simulink model "LagrangeDynamics"  (R2015a)
settings: Solver=ode5  StartTime=0.0  StopTime=10  FixedStep=0.01  RelTol=1e-3
settings Model: Creator=Fares  LastModifiedBy=Fares

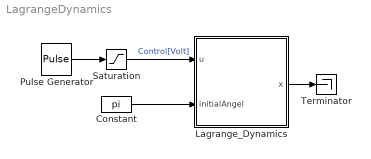
== system LagrangeDynamics ==
  Constant : Constant  Value=pi
  Lagrange_Dynamics : Subsystem  mask{mp=0.95 + 0.025, mc=1.12, l=0.033245968, I=0.013935418, fp=0.000107443, MF=9.4, g=9.81}
      mask prompts: mp "Pedulum mass [kg]"; mc "Cart mass [kg]"; l "Distance from the base to the system CoM [m]"; I "Pendulum of moment of inertia [kg*m2]"; fp "Rotational friction [N ms/rad]"; MF "Maximum Control force [N]"; g "Gravitational acceleration [m/s2]"
      mask init:
      | vf = MF/2.5;
      | M = mc + mp;
      | It = I + mp*l^2;
  Pulse Generator : DiscretePulseGenerator  PulseType=Time based  Period=100  PulseWidth=0.5
  Saturation : Saturate  UpperLimit=2.5  LowerLimit=-2.5
  Terminator : Terminator
  wires:
  Saturation/1 -> Lagrange_Dynamics/1(u)  "Control[Volt]"
  Pulse Generator/1 -> Saturation/1
  Constant/1 -> Lagrange_Dynamics/2(initialAngel)
  Lagrange_Dynamics/1(x) -> Terminator/1

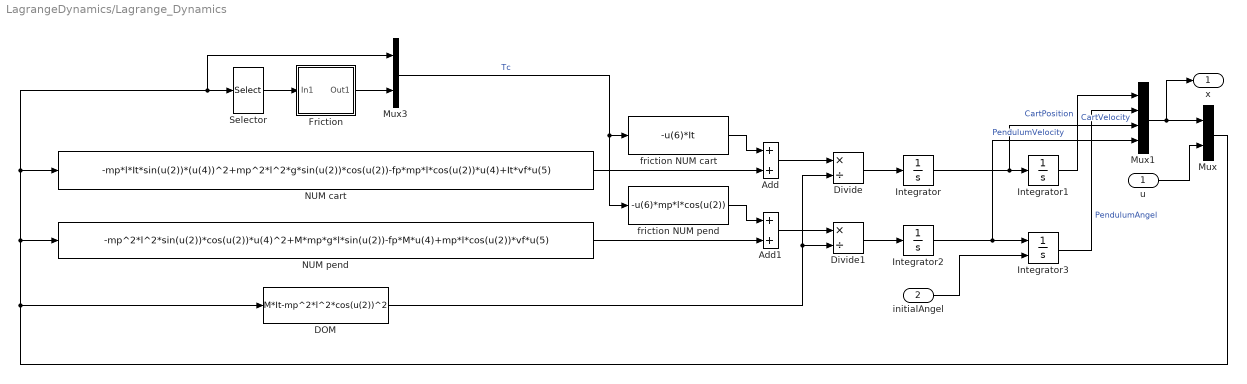
== system LagrangeDynamics/Lagrange_Dynamics ==
  u : Inport
  initialAngel : Inport  Port=2
  Add : Sum
  Add1 : Sum
  "DOM " : Fcn  Expr=M*It-mp^2*l^2*cos(u(2))^2
  Divide : Product  Inputs=*/
  Divide1 : Product  Inputs=*/
  Friction : Subsystem  mask{FS=2.53165, FC=2.28133, DZcv=0.00793711, Xc=0.9, Yc=2.3}
      mask prompts: FS "Static friction [N]"; FC "Coulombic friction [N]"; DZcv "Minimum cart velocity [rad/s]"; Xc "Cart velocity - beginning of the linear dependence zone [m/s]"; Yc "Friction value for Xc point [N]"
      mask init:
      | small = DZcv;
      mask Display: plot([-4 4],[0 0],[-3.8 -2.4 -1.8 -1.2 -0.6 -0.2 0 0.2 0.6 1.2 1.8 2.4 3.8],[-1.4 -1 -1.1 -1.3 -1.6 -2 0 2 1.6 1.3 1.1 1 1.4]);
  Integrator : Integrator
  Integrator1 : Integrator
  Integrator2 : Integrator
  Integrator3 : Integrator  InitialConditionSource=external  InitialCondition=pi
  Mux : Mux  Inputs=2
  Mux1 : Mux
  Mux3 : Mux  Inputs=2
  "NUM cart " : Fcn  Expr=-mp*l*It*sin(u(2))*(u(4))^2+mp^2*l^2*g*sin(u(2))*cos(u(2))-fp*mp*l*cos(u(2))*u(4)+It*vf*u(5)
  NUM pend : Fcn  Expr=-mp^2*l^2*sin(u(2))*cos(u(2))*u(4)^2+M*mp*g*l*sin(u(2))-fp*M*u(4)+mp*l*cos(u(2))*vf*u(5)
  Selector : Selector  InputPortWidth=5  Indices=[3]
  friction NUM cart : Fcn  Expr=-u(6)*It
  friction NUM pend : Fcn  Expr=-u(6)*mp*l*cos(u(2))
  x : Outport
  wires:
  "DOM "/1 -> Divide/2, Divide1/2
  Mux/1 -> Mux3/1, Selector/1, "NUM cart "/1, NUM pend/1, "DOM "/1
  Divide/1 -> Integrator/1
  Integrator2/1 -> Mux1/4, Integrator3/1  "PendulumVelocity"
  u/1 -> Mux/2
  Divide1/1 -> Integrator2/1
  Integrator1/1 -> Mux1/1  "CartPosition"
  Integrator3/1 -> Mux1/2  "PendulumAngel"
  initialAngel/1 -> Integrator3/2
  Integrator/1 -> Mux1/3, Integrator1/1  "CartVelocity"
  Mux1/1 -> x/1, Mux/1
  Selector/1 -> Friction/1(In1)
  "NUM cart "/1 -> Add/2
  NUM pend/1 -> Add1/2
  friction NUM cart/1 -> Add/1
  friction NUM pend/1 -> Add1/1
  Friction/1(Out1) -> Mux3/2
  Mux3/1 -> friction NUM pend/1, friction NUM cart/1  "Tc"
  Add/1 -> Divide/1
  Add1/1 -> Divide1/1

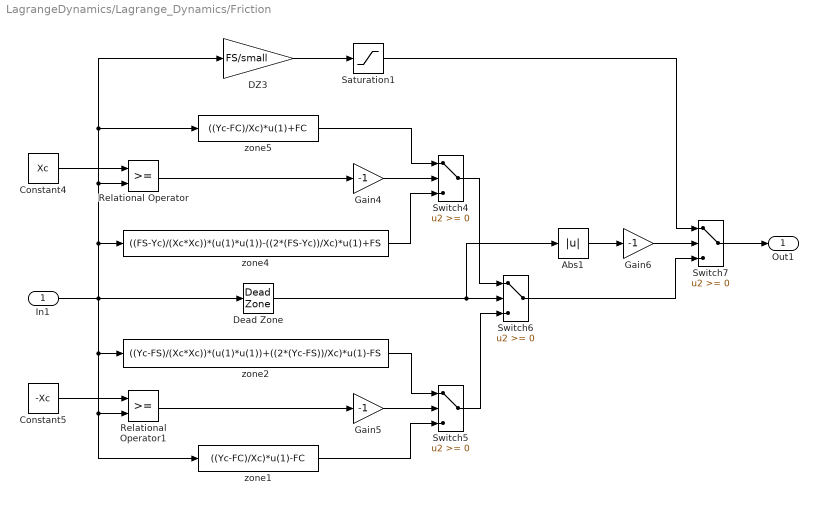
== system LagrangeDynamics/Lagrange_Dynamics/Friction ==
  In1 : Inport
  Abs1 : Abs
  Constant4 : Constant  Value=Xc
  Constant5 : Constant  Value=-Xc
  DZ3 : Gain  Gain=FS/small
  Dead Zone : DeadZone  LowerValue=-DZcv  UpperValue=DZcv  SaturateOnIntegerOverflow=on
  Gain4 : Gain  Gain=-1
  Gain5 : Gain  Gain=-1
  Gain6 : Gain  Gain=-1
  Relational Operator : RelationalOperator  OutDataTypeStr=boolean
  Relational Operator1 : RelationalOperator  OutDataTypeStr=boolean
  Saturation1 : Saturate  UpperLimit=FS  LowerLimit=-FS
  Switch{4..7} (4 alike) : Switch
  zone1 : Fcn  Expr=((Yc-FC)/Xc)*u(1)-FC
  zone2 : Fcn  Expr=((Yc-FS)/(Xc*Xc))*(u(1)*u(1))+((2*(Yc-FS))/Xc)*u(1)-FS
  zone4 : Fcn  Expr=((FS-Yc)/(Xc*Xc))*(u(1)*u(1))-((2*(FS-Yc))/Xc)*u(1)+FS
  zone5 : Fcn  Expr=((Yc-FC)/Xc)*u(1)+FC
  Out1 : Outport
  wires:
  Gain4/1 -> Switch4/2
  Dead Zone/1 -> Abs1/1, Switch6/2
  Gain5/1 -> Switch5/2
  Relational Operator/1 -> Gain4/1
  Constant5/1 -> Relational Operator1/1
  Relational Operator1/1 -> Gain5/1
  Abs1/1 -> Gain6/1
  DZ3/1 -> Saturation1/1
  Switch6/1 -> Switch7/3
  Switch4/1 -> Switch6/1
  zone2/1 -> Switch5/1
  Gain6/1 -> Switch7/2
  zone4/1 -> Switch4/3
  Switch7/1 -> Out1/1
  In1/1 -> zone1/1, Relational Operator1/2, zone2/1, DZ3/1, zone5/1, Relational Operator/2, zone4/1, Dead Zone/1
  Saturation1/1 -> Switch7/1
  zone5/1 -> Switch4/1
  Constant4/1 -> Relational Operator/1
  zone1/1 -> Switch5/3
  Switch5/1 -> Switch6/3
